simulink model "StSys_StrtCtl"  (R2016b)
settings: configuration reference "CodeGenConfigSet" (kept outside this file)
values from neighbouring files (symbols this model uses):
  Strt_uThresIniMinStrt_C = Calibration.Parameter    [init_StSys_StrtCtl.m]    (also in init_StSys_StrtCtl_SIL.m = Simulink.Parameter)
  StSys_nBlnd_C = Calibration.Parameter    [init_StSys_StrtCtl.m]    (also in init_StSys_StrtCtl_SIL.m = Simulink.Parameter)
  StSys_nThres_C = Calibration.Parameter    [init_StSys_StrtCtl.m]    (also in init_StSys_StrtCtl_SIL.m = Simulink.Parameter)
  StSys_nThresCalc_CUR = Calibration.Parameter    [init_StSys_StrtCtl.m]    (also in init_StSys_StrtCtl_SIL.m = Simulink.Parameter)
  StSys_nThresCalc_CURX = Calibration.Parameter    [init_StSys_StrtCtl.m]    (also in init_StSys_StrtCtl_SIL.m = Simulink.Parameter)
  StSys_stCondActv_C = Calibration.Parameter    [init_StSys_StrtCtl.m]    (also in init_StSys_StrtCtl_SIL.m = Simulink.Parameter)
  StSys_stCondDeactv_C = Calibration.Parameter    [init_StSys_StrtCtl.m]    (also in init_StSys_StrtCtl_SIL.m = Simulink.Parameter)
  StSys_stLogicT50CAN_C = Calibration.Parameter    [init_StSys_StrtCtl.m]    (also in init_StSys_StrtCtl_SIL.m = Simulink.Parameter)
  StSys_stLogicT50EMGCY_C = Calibration.Parameter    [init_StSys_StrtCtl.m]    (also in init_StSys_StrtCtl_SIL.m = Simulink.Parameter)
  StSys_stLogicT50NRM_C = Calibration.Parameter    [init_StSys_StrtCtl.m]    (also in init_StSys_StrtCtl_SIL.m = Simulink.Parameter)
  StSys_stSelectT50CAN_C = Calibration.Parameter    [init_StSys_StrtCtl.m]    (also in init_StSys_StrtCtl_SIL.m = Simulink.Parameter)
  StSys_stSelectT50EMGCY_C = Calibration.Parameter    [init_StSys_StrtCtl.m]    (also in init_StSys_StrtCtl_SIL.m = Simulink.Parameter)
  StSys_stSelectT50NRM_C = Calibration.Parameter    [init_StSys_StrtCtl.m]    (also in init_StSys_StrtCtl_SIL.m = Simulink.Parameter)
  StSys_tiBlnd_C = Calibration.Parameter    [init_StSys_StrtCtl.m]    (also in init_StSys_StrtCtl_SIL.m = Simulink.Parameter)
  StSys_tiStrtON_C = Calibration.Parameter    [init_StSys_StrtCtl.m]    (also in init_StSys_StrtCtl_SIL.m = Simulink.Parameter)
  StSys_vEngCompStrt_C = Calibration.Parameter    [init_StSys_StrtCtl.m]    (also in init_StSys_StrtCtl_SIL.m = Simulink.Parameter)
  StSys_vThresT50CAN_C = Calibration.Parameter    [init_StSys_StrtCtl.m]    (also in init_StSys_StrtCtl_SIL.m = Simulink.Parameter)
  StSys_vThresT50EMGCY_C = Calibration.Parameter    [init_StSys_StrtCtl.m]    (also in init_StSys_StrtCtl_SIL.m = Simulink.Parameter)
  StSys_vThresT50NRM_C = Calibration.Parameter    [init_StSys_StrtCtl.m]    (also in init_StSys_StrtCtl_SIL.m = Simulink.Parameter)
undefined symbols (not defined in the file or in its folder): AirHtState_conv, StSys_StrtCtl_DT, StSys_StrtState_conv
libraries: simulink x201, CXLib x7
(part 1 of 2)
settings Model: Creator=xuxingpei  LastModifiedBy=xuxingpei
settings ConfigSetRef: SourceLocation=Base Workspace

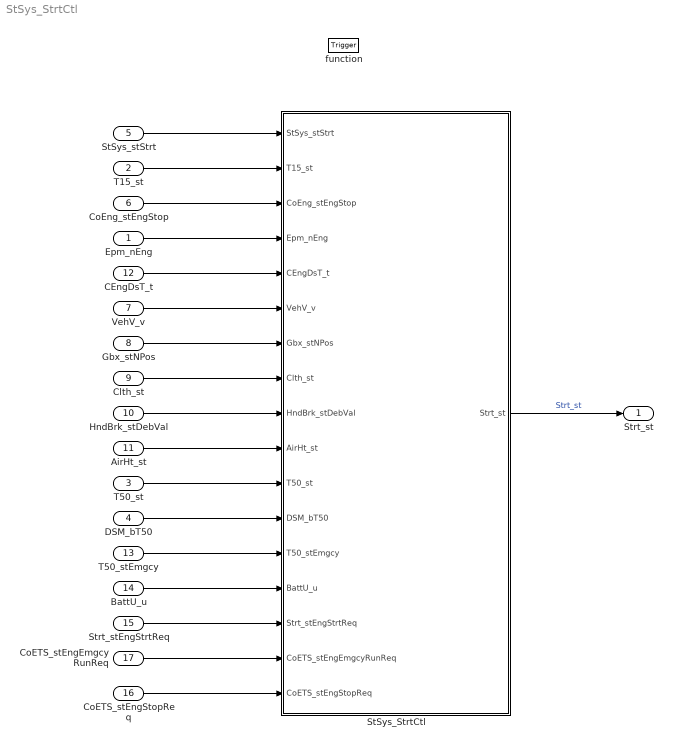
== system StSys_StrtCtl ==
  Epm_nEng : Inport  Tag=rpm  Description=Engine speed  OutMin=0  OutMax=6000  OutDataTypeStr=EngSpeed_rpm
  T15_st : Inport  Description=Terminal 15 status after debouncing  Port=2  OutDataTypeStr=Enum: Switch_conv
  T50_st : Inport  Description=Terminal 50 status after debouncing  Port=3  OutDataTypeStr=Enum: Switch_conv
  DSM_bT50 : Inport  Description=DSM status from T50 switch  Port=4  OutMin=0  OutMax=1  OutDataTypeStr=boolean
  StSys_stStrt : Inport  Description=state of starting system  Port=5  OutDataTypeStr=Enum: StSys_StrtState_conv
  CoEng_stEngStop : Inport  Description=Bit coded output message from engine stop function for low idle, egine shut off and crank control  Port=6  OutMin=0  OutMax=255  OutDataTypeStr=State_uint8
  VehV_v : Inport  Tag=km/h  Description=Vehicle speed  Port=7  OutMin=0  OutMax=250  OutDataTypeStr=VehSpeed_km_h
  Gbx_stNPos : Inport  Description=Gearbox neutral position status signal  Port=8  OutMin=0  OutMax=255  OutDataTypeStr=State_uint8
  Clth_st : Inport  Description=Clutch information  Port=9  OutMin=0  OutMax=255  OutDataTypeStr=State_uint8
  HndBrk_stDebVal : Inport  Description=Debounced value of Hand Brake switch  Port=10  OutMin=0  OutMax=255  OutDataTypeStr=State_uint8
  AirHt_st : Inport  Description=status of AirHeater  Port=11  OutDataTypeStr=Enum: AirHtState_conv
  CEngDsT_t : Inport  Tag=deg  Description=Coolant engine down stream temperature  Port=12  OutMin=-200  OutMax=200  OutDataTypeStr=Temp_deg
  T50_stEmgcy : Inport  Description=Terminal 50 status after debouncing  Port=13  OutMin=0  OutMax=1  OutDataTypeStr=boolean
  BattU_u : Inport  Tag=mv  Description=Battery voltage  Port=14  OutMin=0  OutMax=50000  OutDataTypeStr=Battery_mv
  Strt_stEngStrtReq : Inport  Description=start switch via CAN  Port=15  OutMin=0  OutMax=1  OutDataTypeStr=boolean
  CoETS_stEngStopReq : Inport  Description=Tbox Engine stop request  Port=16  OutMin=0  OutMax=1  OutDataTypeStr=boolean
  CoETS_stEngEmgcyRunReq : Inport  Description=Tbox Engine emergency start request  Port=17  OutMin=0  OutMax=1  OutDataTypeStr=boolean
  function : TriggerPort  TriggerType=function-call  VariantControl=Variant
  StSys_StrtCtl : Subsystem
  Strt_st : Outport  Description=Control signal for the starter relay  OutMin=0  OutMax=1  OutDataTypeStr=boolean
  wires:
  StSys_stStrt/1 -> StSys_StrtCtl/1(StSys_stStrt)
  T15_st/1 -> StSys_StrtCtl/2(T15_st)
  CoEng_stEngStop/1 -> StSys_StrtCtl/3(CoEng_stEngStop)
  Epm_nEng/1 -> StSys_StrtCtl/4(Epm_nEng)
  CEngDsT_t/1 -> StSys_StrtCtl/5(CEngDsT_t)
  VehV_v/1 -> StSys_StrtCtl/6(VehV_v)
  Gbx_stNPos/1 -> StSys_StrtCtl/7(Gbx_stNPos)
  Clth_st/1 -> StSys_StrtCtl/8(Clth_st)
  HndBrk_stDebVal/1 -> StSys_StrtCtl/9(HndBrk_stDebVal)
  AirHt_st/1 -> StSys_StrtCtl/10(AirHt_st)
  T50_st/1 -> StSys_StrtCtl/11(T50_st)
  DSM_bT50/1 -> StSys_StrtCtl/12(DSM_bT50)
  StSys_StrtCtl/1(Strt_st) -> Strt_st/1  "Strt_st"
  T50_stEmgcy/1 -> StSys_StrtCtl/13(T50_stEmgcy)
  BattU_u/1 -> StSys_StrtCtl/14(BattU_u)
  Strt_stEngStrtReq/1 -> StSys_StrtCtl/15(Strt_stEngStrtReq)
  CoETS_stEngStopReq/1 -> StSys_StrtCtl/17(CoETS_stEngStopReq)
  CoETS_stEngEmgcyRunReq/1 -> StSys_StrtCtl/16(CoETS_stEngEmgcyRunReq)

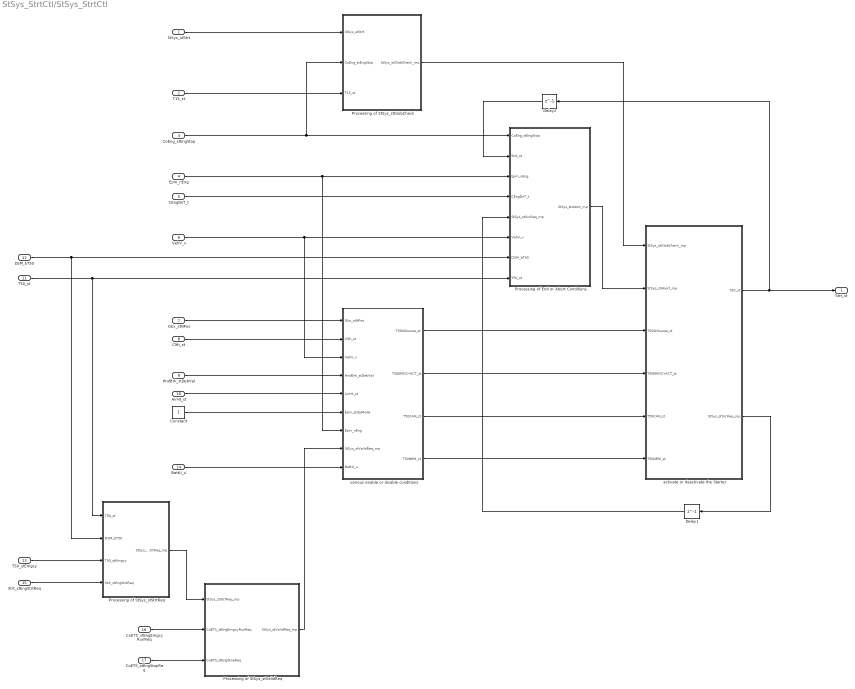
== system StSys_StrtCtl/StSys_StrtCtl ==
  StSys_stStrt : Inport  Description=state of starting system  OutDataTypeStr=Enum: StSys_StrtState_conv
  T15_st : Inport  Description=Terminal 15 status after debouncing  Port=2  OutDataTypeStr=Enum: Switch_conv
  CoEng_stEngStop : Inport  Description=Bit coded output message from engine stop function for low idle, egine shut off and crank control  Port=3  OutMin=0  OutMax=255  OutDataTypeStr=State_uint8
  Epm_nEng : Inport  Tag=rpm  Description=Engine speed  Port=4  OutMin=0  OutMax=6000  OutDataTypeStr=EngSpeed_rpm
  CEngDsT_t : Inport  Tag=deg  Description=Coolant engine down stream temperature  Port=5  OutMin=-200  OutMax=200  OutDataTypeStr=Temp_deg
  VehV_v : Inport  Tag=km/h  Description=Vehicle speed  Port=6  OutMin=0  OutMax=250  OutDataTypeStr=VehSpeed_km_h
  Gbx_stNPos : Inport  Description=Gearbox neutral position status signal  Port=7  OutMin=0  OutMax=255  OutDataTypeStr=State_uint8
  Clth_st : Inport  Description=Clutch information  Port=8  OutMin=0  OutMax=255  OutDataTypeStr=State_uint8
  HndBrk_stDebVal : Inport  Description=Debounced value of Hand Brake switch  Port=9  OutMin=0  OutMax=255  OutDataTypeStr=State_uint8
  AirHt_st : Inport  Description=status of AirHeater  Port=10  OutDataTypeStr=Enum: AirHtState_conv
  T50_st : Inport  Description=Terminal 15 status after debouncing  Port=11  OutDataTypeStr=Enum: Switch_conv
  DSM_bT50 : Inport  Description=DSM status from T50 switch  Port=12  OutMin=0  OutMax=1  OutDataTypeStr=boolean
  T50_stEmgcy : Inport  Port=13
  BattU_u : Inport  Port=14
  Strt_stEngStrtReq : Inport  Description=start switch via CAN  Port=15  OutMin=0  OutMax=1  OutDataTypeStr=boolean
  CoETS_stEngEmgcyRunReq : Inport  Port=16
  CoETS_stEngStopReq : Inport  Port=17
  Constant : Constant  OutDataTypeStr=boolean
  Delay1 : Delay  DelayLength=1  InitialCondition=0
  Delay2 : Delay  DelayLength=1  InitialCondition=0
  Processing of End or Abort Conditions : Subsystem
  Processing of StSys_stGlobCheck : Subsystem
  Processing of StSys_stStrtReq : Subsystem
  Processing of StSys_stValidReq : Subsystem
  activate or deactivate the Starter : Subsystem
  various enable or disable conditions : Subsystem
  Strt_st : Outport  Description=Control signal for the starter relay  OutMin=0  OutMax=1  OutDataTypeStr=boolean
  wires:
  activate or deactivate the Starter/1(Strt_st) -> Delay2/1, Strt_st/1
  CoEng_stEngStop/1 -> Processing of StSys_stGlobCheck/2(CoEng_stEngStop), Processing of End or Abort Conditions/1(CoEng_stEngStop)
  Constant/1 -> various enable or disable conditions/6(Epm_stOpMode)
  DSM_bT50/1 -> Processing of StSys_stStrtReq/2(DSM_bT50), Processing of End or Abort Conditions/7(DSM_bT50)
  Processing of StSys_stStrtReq/1(StSys_stStrtReq_mp) -> Processing of StSys_stValidReq/1(StSys_stStrtReq_mp)
  Epm_nEng/1 -> various enable or disable conditions/7(Epm_nEng), Processing of End or Abort Conditions/3(Epm_nEng)
  T50_stEmgcy/1 -> Processing of StSys_stStrtReq/3(T50_stEmgcy)
  HndBrk_stDebVal/1 -> various enable or disable conditions/4(HndBrk_stDebVal)
  StSys_stStrt/1 -> Processing of StSys_stGlobCheck/1(StSys_stStrt)
  Gbx_stNPos/1 -> various enable or disable conditions/1(Gbx_stNPos)
  T50_st/1 -> Processing of StSys_stStrtReq/1(T50_st), Processing of End or Abort Conditions/8(T50_st)
  AirHt_st/1 -> various enable or disable conditions/5(AirHt_st)
  Clth_st/1 -> various enable or disable conditions/2(Clth_st)
  Processing of StSys_stValidReq/1(StSys_stValidReq_mp) -> various enable or disable conditions/8(StSys_stValidReq_mp)
  various enable or disable conditions/1(T50StSourse_st) -> activate or deactivate the Starter/3(T50StSourse_st)
  T15_st/1 -> Processing of StSys_stGlobCheck/3(T15_st)
  VehV_v/1 -> various enable or disable conditions/3(VehV_v), Processing of End or Abort Conditions/6(VehV_v)
  CEngDsT_t/1 -> Processing of End or Abort Conditions/4(CEngDsT_t)
  BattU_u/1 -> various enable or disable conditions/9(BattU_u)
  various enable or disable conditions/2(T50EMGCYACT_st) -> activate or deactivate the Starter/4(T50EMGCYACT_st)
  Processing of StSys_stGlobCheck/1(StSys_stGlobCheck_mp) -> activate or deactivate the Starter/1(StSys_stGlobCheck_mp)
  Processing of End or Abort Conditions/1(StSys_stAbort_mp) -> activate or deactivate the Starter/2(StSys_stAbort_mp)
  activate or deactivate the Starter/2(StSys_stSrcReq_mp) -> Delay1/1
  Delay1/1 -> Processing of End or Abort Conditions/5(StSys_stSrcReq_mp)
  Delay2/1 -> Processing of End or Abort Conditions/2(Strt_st)
  various enable or disable conditions/3(T50CAN_st) -> activate or deactivate the Starter/5(T50CAN_st)
  Strt_stEngStrtReq/1 -> Processing of StSys_stStrtReq/4(Strt_stEngStrtReq)
  various enable or disable conditions/4(T50NRM_st) -> activate or deactivate the Starter/6(T50NRM_st)
  CoETS_stEngEmgcyRunReq/1 -> Processing of StSys_stValidReq/2(CoETS_stEngEmgcyRunReq)
  CoETS_stEngStopReq/1 -> Processing of StSys_stValidReq/3(CoETS_stEngStopReq)

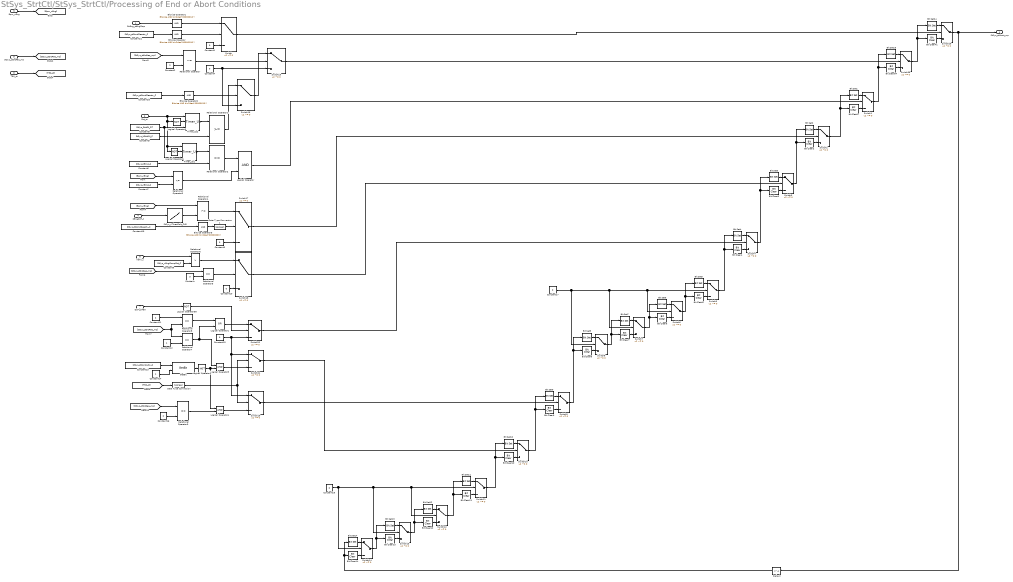
== system StSys_StrtCtl/StSys_StrtCtl/Processing of End or Abort Conditions ==
  CoEng_stEngStop : Inport
  Strt_st : Inport  Port=2
  Epm_nEng : Inport  Port=3
  CEngDsT_t : Inport  Port=4
  StSys_stSrcReq_mp : Inport  Port=5
  VehV_v : Inport  Port=6
  DSM_bT50 : Inport  Port=7
  T50_st : Inport  Port=8
  Bit Clear1 : simulink/Logic and Bit Operations/Bit Clear  iBit=2
  Bit Clear10 : simulink/Logic and Bit Operations/Bit Clear  iBit=11
  Bit Clear11 : simulink/Logic and Bit Operations/Bit Clear  iBit=12
  Bit Clear12 : simulink/Logic and Bit Operations/Bit Clear  iBit=13
  Bit Clear13 : simulink/Logic and Bit Operations/Bit Clear  iBit=14
  Bit Clear14 : simulink/Logic and Bit Operations/Bit Clear  iBit=15
  Bit Clear2 : simulink/Logic and Bit Operations/Bit Clear  iBit=3
  Bit Clear3 : simulink/Logic and Bit Operations/Bit Clear  iBit=4
  Bit Clear4 : simulink/Logic and Bit Operations/Bit Clear  iBit=5
  Bit Clear41 : simulink/Logic and Bit Operations/Bit Clear  iBit=0
  Bit Clear5 : simulink/Logic and Bit Operations/Bit Clear  iBit=6
  Bit Clear54 : simulink/Logic and Bit Operations/Bit Clear  iBit=1
  Bit Clear6 : simulink/Logic and Bit Operations/Bit Clear  iBit=7
  Bit Clear7 : simulink/Logic and Bit Operations/Bit Clear  iBit=8
  Bit Clear8 : simulink/Logic and Bit Operations/Bit Clear  iBit=9
  Bit Clear9 : simulink/Logic and Bit Operations/Bit Clear  iBit=10
  Bit Set1 : simulink/Logic and Bit Operations/Bit Set  iBit=2
  Bit Set10 : simulink/Logic and Bit Operations/Bit Set  iBit=11
  Bit Set11 : simulink/Logic and Bit Operations/Bit Set  iBit=12
  Bit Set12 : simulink/Logic and Bit Operations/Bit Set  iBit=13
  Bit Set13 : simulink/Logic and Bit Operations/Bit Set  iBit=14
  Bit Set14 : simulink/Logic and Bit Operations/Bit Set  iBit=15
  Bit Set18 : simulink/Logic and Bit Operations/Bit Set  iBit=1
  Bit Set2 : simulink/Logic and Bit Operations/Bit Set  iBit=3
  Bit Set24 : simulink/Logic and Bit Operations/Bit Set  iBit=0
  Bit Set3 : simulink/Logic and Bit Operations/Bit Set  iBit=4
  Bit Set4 : simulink/Logic and Bit Operations/Bit Set  iBit=5
  Bit Set5 : simulink/Logic and Bit Operations/Bit Set  iBit=6
  Bit Set6 : simulink/Logic and Bit Operations/Bit Set  iBit=7
  Bit Set7 : simulink/Logic and Bit Operations/Bit Set  iBit=8
  Bit Set8 : simulink/Logic and Bit Operations/Bit Set  iBit=9
  Bit Set9 : simulink/Logic and Bit Operations/Bit Set  iBit=10
  Bitwise Operator : simulink/Logic and Bit Operations/Bitwise Operator  logicop=AND  UseBitMask=on  BitMask=bin2dec('00000100')  BitMaskRealWorld=Stored Integer
  Bitwise Operator1 : simulink/Logic and Bit Operations/Bitwise Operator  logicop=AND  UseBitMask=on  BitMask=bin2dec('00000010')  BitMaskRealWorld=Stored Integer
  Bitwise Operator2 : simulink/Logic and Bit Operations/Bitwise Operator  logicop=AND  UseBitMask=on  BitMask=bin2dec('00000010')  BitMaskRealWorld=Stored Integer
  Bitwise Operator3 : simulink/Logic and Bit Operations/Bitwise Operator  logicop=AND  UseBitMask=on  BitMask=bin2dec('00000001')  BitMaskRealWorld=Stored Integer
  Constant : Constant  Value=3  OutDataTypeStr=Inherit: Inherit via back propagation
  Constant{1,3..4,10,15} (5 alike) : Constant  Value=0  OutDataTypeStr=Inherit: Inherit via back propagation
  Constant11 : Constant  Value=2  OutDataTypeStr=Inherit: Inherit via back propagation
  Constant12 : Constant  OutDataTypeStr=Inherit: Inherit via back propagation
  Constant13 : Constant  Value=StSys_stCondActv_C
  Constant14 : Constant  OutDataTypeStr=Inherit: Inherit via back propagation
  Constant16 : Constant  Value=2  OutDataTypeStr=Inherit: Inherit via back propagation
  Constant17 : Constant  Value=0  OutDataTypeStr=boolean
  Constant18 : Constant  Value=0  OutDataTypeStr=boolean
  Constant19 : Constant  Value=StSys_stCondDeactv_C
  Constant2 : Constant  Value=2  OutDataTypeStr=Inherit: Inherit via back propagation
  Constant20 : Constant  Value=StSys_stCondDeactv_C
  Constant21 : Constant  Value=StSys_stCondDeactv_C
  Constant5 : Constant  Value=StSys_tiStrtON_C
  Constant6 : Constant  Value=StSys_tiBlnd_C
  Constant7 : Constant  Value=StSys_nBlnd_C
  Constant8 : Constant  Value=StSys_StrtCtl_DT
  Constant9 : Constant  Value=StSys_vEngCompStrt_C
  Data Type Conversion : DataTypeConversion  OutDataTypeStr=boolean
  Data Type Conversion1 : DataTypeConversion  OutDataTypeStr=boolean
  Delay2 : Delay  DelayLength=1  InitialCondition=0
  GetBit : CXLib/GetBit  dataTypeString=uint16  dataLength=0
      settings: AttributesFormatString=Get bit from %<dataTypeString>
  Logical Operator : Logic  OutDataTypeStr=boolean
  Logical Operator1 : Logic  Operator=OR  AllPortsSameDT=off  OutDataTypeStr=boolean
  Logical Operator{2,5..6,38} (4 alike) : Logic  Operator=NOT  AllPortsSameDT=off  OutDataTypeStr=boolean
  Logical Operator3 : Logic  AllPortsSameDT=off  OutDataTypeStr=boolean
  Logical Operator4 : Logic  AllPortsSameDT=off  OutDataTypeStr=boolean
  Relational Operator : RelationalOperator  Operator=~=  OutDataTypeStr=boolean  RndMeth=Simplest  InputSameDT=on
  Relational Operator1 : RelationalOperator  OutDataTypeStr=boolean  RndMeth=Simplest
  Relational Operator2 : RelationalOperator  OutDataTypeStr=boolean  RndMeth=Simplest
  Relational Operator3 : RelationalOperator  Operator=<=  OutDataTypeStr=boolean  RndMeth=Simplest
  Relational Operator4 : RelationalOperator  OutDataTypeStr=boolean  RndMeth=Simplest
  Relational Operator{5,7..9} (4 alike) : RelationalOperator  Operator===  OutDataTypeStr=boolean  RndMeth=Simplest  InputSameDT=on
  Relational Operator6 : RelationalOperator  Operator=>  OutDataTypeStr=boolean  RndMeth=Simplest
  StSys_nThresCalc_CUR : Lookup_n-D  NumberOfTableDimensions=1  BreakpointsForDimension1=StSys_nThresCalc_CURX  BreakpointsForDimension1DataTypeStr=Temp_deg  IndexSearchMethod=Linear search  Table=StSys_nThresCalc_CUR  TableDataTypeStr=EngSpeed_rpm  ExtrapMethod=Clip  InternalRulePriority=Speed  OutDataTypeStr=EngSpeed_rpm  RndMeth=Simplest  InputSameDT=on
  Switch{,1..14,16..18,20,29,36} (21 alike) : Switch  Criteria=u2 ~= 0  InputSameDT=on
  Switch15 : Switch  Criteria=u2 ~= 0
  Switch19 : Switch  Criteria=u2 ~= 0
  Switch21 : Switch  Criteria=u2 ~= 0
  Timer_Up1 : CXLib/Timer_Up
  Timer_Up2 : CXLib/Timer_Up
  StSys_stAbort_mp : Outport
  wires:
  Switch29/1 -> Delay2/1, StSys_stAbort_mp/1  "StSys_stAbort_mp"
  Bit Set24/1 -> Switch29/1
  Bit Clear41/1 -> Switch29/3
  Delay2/1 -> Bit Clear14/1, Bit Set14/1
  Switch36/1 -> Bit Clear41/1, Bit Set24/1
  Bit Set18/1 -> Switch36/1
  Bit Clear54/1 -> Switch36/3
  Switch1/1 -> Bit Set18/1, Bit Clear54/1
  Bit Set1/1 -> Switch1/1
  Bit Clear1/1 -> Switch1/3
  Switch2/1 -> Bit Set1/1, Bit Clear1/1
  Bit Set2/1 -> Switch2/1
  Bit Clear2/1 -> Switch2/3
  Switch3/1 -> Bit Clear2/1, Bit Set2/1
  Bit Set3/1 -> Switch3/1
  Bit Clear3/1 -> Switch3/3
  Switch4/1 -> Bit Set3/1, Bit Clear3/1
  Bit Set4/1 -> Switch4/1
  Bit Clear4/1 -> Switch4/3
  Switch5/1 -> Bit Set4/1, Bit Clear4/1
  Bit Set5/1 -> Switch5/1
  Bit Clear5/1 -> Switch5/3
  Switch6/1 -> Bit Set5/1, Bit Clear5/1
  Bit Set6/1 -> Switch6/1
  Bit Clear6/1 -> Switch6/3
  Switch7/1 -> Bit Set6/1, Bit Clear6/1
  Bit Set7/1 -> Switch7/1
  Bit Clear7/1 -> Switch7/3
  Switch8/1 -> Bit Set7/1, Bit Clear7/1
  Bit Set8/1 -> Switch8/1
  Bit Clear8/1 -> Switch8/3
  Switch9/1 -> Bit Set8/1, Bit Clear8/1
  Bit Set9/1 -> Switch9/1
  Bit Clear9/1 -> Switch9/3
  Switch10/1 -> Bit Set9/1, Bit Clear9/1
  Bit Set10/1 -> Switch10/1
  Bit Clear10/1 -> Switch10/3
  Switch11/1 -> Bit Clear10/1, Bit Set10/1
  Bit Set11/1 -> Switch11/1
  Bit Clear11/1 -> Switch11/3
  Switch12/1 -> Bit Set11/1, Bit Clear11/1
  Bit Set12/1 -> Switch12/1
  Bit Clear12/1 -> Switch12/3
  Switch13/1 -> Bit Set12/1, Bit Clear12/1
  Bit Set13/1 -> Switch13/1
  Bit Clear13/1 -> Switch13/3
  Switch14/1 -> Bit Set13/1, Bit Clear13/1
  Bit Set14/1 -> Switch14/1
  Bit Clear14/1 -> Switch14/3
  Bitwise Operator/1 -> Switch/2
  CoEng_stEngStop/1 -> Bitwise Operator1/1
  Constant21/1 -> Bitwise Operator/1
  [StSys_stSrcReq_mp] -> Relational Operator/1
  Constant2/1 -> Relational Operator/2
  Relational Operator/1 -> Switch15/2
  Constant20/1 -> Bitwise Operator2/1
  Bitwise Operator2/1 -> Switch16/2
  Constant4/1 -> Switch16/3, Switch15/3
  Timer_Up1/1 -> Relational Operator2/1
  Constant6/1 -> Relational Operator2/2
  Timer_Up2/1 -> Relational Operator1/1
  Constant5/1 -> Relational Operator1/2
  [Epm_nEng] -> Relational Operator3/1
  Constant7/1 -> Relational Operator3/2
  Relational Operator2/1 -> Logical Operator/1
  Relational Operator3/1 -> Logical Operator/2
  Epm_nEng/1 -> [Epm_nEng]
  Constant19/1 -> Bitwise Operator3/1
  CEngDsT_t/1 -> StSys_nThresCalc_CUR/1
  StSys_nThresCalc_CUR/1 -> Relational Operator4/2
  [Epm_nEng] -> Relational Operator4/1
  Bitwise Operator3/1 -> Data Type Conversion1/1
  StSys_stSrcReq_mp/1 -> [StSys_stSrcReq_mp]
  [StSys_stSrcReq_mp] -> Relational Operator5/1
  Constant/1 -> Relational Operator5/2
  VehV_v/1 -> Relational Operator6/1
  Constant9/1 -> Relational Operator6/2
  Relational Operator5/1 -> Switch18/2
  DSM_bT50/1 -> Logical Operator38/1
  Logical Operator38/1 -> Switch20/2
  Relational Operator8/1 -> Logical Operator1/1
  Relational Operator7/1 -> Logical Operator1/2, Logical Operator3/1
  [StSys_stSrcReq_mp] -> Relational Operator8/2, Relational Operator7/1
  Constant11/1 -> Relational Operator8/1
  Constant12/1 -> Relational Operator7/2
  Constant13/1 -> GetBit/1
  Constant14/1 -> GetBit/2
  GetBit/1 -> Logical Operator2/1
  Logical Operator2/1 -> Logical Operator4/1, Logical Operator3/2
  T50_st/1 -> [T50_st]
  [T50_st] -> Data Type Conversion/1
  Constant15/1 -> Switch19/1, Switch21/1, Switch20/3
  [StSys_stSrcReq_mp] -> Relational Operator9/1
  Constant16/1 -> Relational Operator9/2
  Relational Operator9/1 -> Logical Operator4/2
  Switch/1 -> Switch29/2
  Switch15/1 -> Switch36/2
  Logical Operator/1 -> Switch1/2
  Constant17/1 -> Switch8/2, Switch7/2, Switch6/2, Switch5/2
  Constant18/1 -> Switch14/2, Switch13/2, Switch12/2, Switch11/2
  Switch21/1 -> Switch10/2
  Switch19/1 -> Switch9/2
  Constant8/1 -> Timer_Up2/3, Timer_Up1/3
  Switch17/1 -> Switch2/2
  Switch18/1 -> Switch3/2
  Switch20/1 -> Switch4/2
  Logical Operator4/1 -> Switch19/3
  Logical Operator3/1 -> Switch21/3
  Logical Operator1/1 -> Switch20/1
  Relational Operator6/1 -> Switch18/1
  Constant10/1 -> Switch18/3
  Relational Operator4/1 -> Switch17/1
  Constant3/1 -> Switch17/3
  Relational Operator1/1 -> Switch16/1
  Switch16/1 -> Switch15/1
  Bitwise Operator1/1 -> Switch/1
  Constant1/1 -> Switch/3
  Data Type Conversion/1 -> Switch19/2, Switch21/2
  Data Type Conversion1/1 -> Switch17/2
  Logical Operator5/1 -> Timer_Up2/2
  Logical Operator6/1 -> Timer_Up1/2
  Strt_st/1 -> Timer_Up2/1, Logical Operator5/1, Logical Operator6/1, Timer_Up1/1

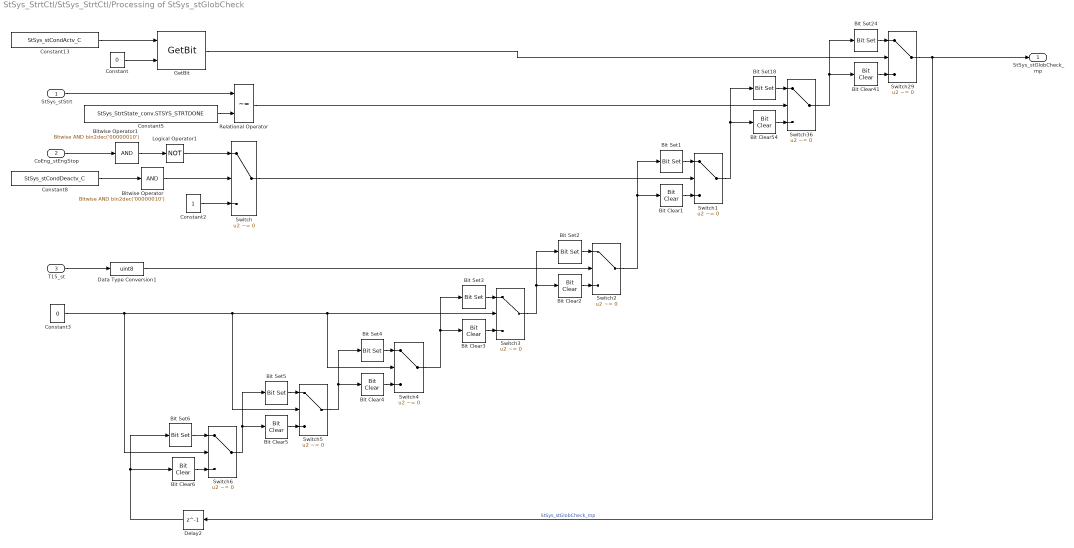
== system StSys_StrtCtl/StSys_StrtCtl/Processing of StSys_stGlobCheck ==
  StSys_stStrt : Inport
  CoEng_stEngStop : Inport  Port=2
  T15_st : Inport  Port=3
  Bit Clear1 : simulink/Logic and Bit Operations/Bit Clear  iBit=2
  Bit Clear2 : simulink/Logic and Bit Operations/Bit Clear  iBit=3
  Bit Clear3 : simulink/Logic and Bit Operations/Bit Clear  iBit=4
  Bit Clear4 : simulink/Logic and Bit Operations/Bit Clear  iBit=5
  Bit Clear41 : simulink/Logic and Bit Operations/Bit Clear  iBit=0
  Bit Clear5 : simulink/Logic and Bit Operations/Bit Clear  iBit=6
  Bit Clear54 : simulink/Logic and Bit Operations/Bit Clear  iBit=1
  Bit Clear6 : simulink/Logic and Bit Operations/Bit Clear  iBit=7
  Bit Set1 : simulink/Logic and Bit Operations/Bit Set  iBit=2
  Bit Set18 : simulink/Logic and Bit Operations/Bit Set  iBit=1
  Bit Set2 : simulink/Logic and Bit Operations/Bit Set  iBit=3
  Bit Set24 : simulink/Logic and Bit Operations/Bit Set  iBit=0
  Bit Set3 : simulink/Logic and Bit Operations/Bit Set  iBit=4
  Bit Set4 : simulink/Logic and Bit Operations/Bit Set  iBit=5
  Bit Set5 : simulink/Logic and Bit Operations/Bit Set  iBit=6
  Bit Set6 : simulink/Logic and Bit Operations/Bit Set  iBit=7
  Bitwise Operator : simulink/Logic and Bit Operations/Bitwise Operator  logicop=AND  UseBitMask=on  BitMask=bin2dec('00000010')  BitMaskRealWorld=Stored Integer
  Bitwise Operator1 : simulink/Logic and Bit Operations/Bitwise Operator  logicop=AND  UseBitMask=on  BitMask=bin2dec('00000010')  BitMaskRealWorld=Stored Integer
  Constant : Constant  Value=0  OutDataTypeStr=uint8
  Constant13 : Constant  Value=StSys_stCondActv_C
  Constant2 : Constant  OutDataTypeStr=Inherit: Inherit via back propagation
  Constant3 : Constant  Value=0  OutDataTypeStr=boolean
  Constant5 : Constant  Value=StSys_StrtState_conv.STSYS_STRTDONE
  Constant8 : Constant  Value=StSys_stCondDeactv_C
  Data Type Conversion1 : DataTypeConversion  OutDataTypeStr=uint8
  Delay2 : Delay  DelayLength=1  InitialCondition=0
  GetBit : CXLib/GetBit  dataTypeString=uint16  dataLength=0
      settings: AttributesFormatString=Get bit from %<dataTypeString>
  Logical Operator1 : Logic  Operator=NOT  AllPortsSameDT=off  OutDataTypeStr=boolean
  Relational Operator : RelationalOperator  Operator=~=  OutDataTypeStr=boolean  RndMeth=Simplest
  Switch{,1..6,29,36} (9 alike) : Switch  Criteria=u2 ~= 0  InputSameDT=on
  StSys_stGlobCheck_mp : Outport
  wires:
  Switch29/1 -> StSys_stGlobCheck_mp/1, Delay2/1  "StSys_stGlobCheck_mp"
  Bit Set24/1 -> Switch29/1
  Bit Clear41/1 -> Switch29/3
  Switch36/1 -> Bit Clear41/1, Bit Set24/1
  Bit Set18/1 -> Switch36/1
  Bit Clear54/1 -> Switch36/3
  Switch1/1 -> Bit Set18/1, Bit Clear54/1
  Bit Set1/1 -> Switch1/1
  Bit Clear1/1 -> Switch1/3
  Switch2/1 -> Bit Set1/1, Bit Clear1/1
  Bit Set2/1 -> Switch2/1
  Bit Clear2/1 -> Switch2/3
  Switch3/1 -> Bit Clear2/1, Bit Set2/1
  Bit Set3/1 -> Switch3/1
  Bit Clear3/1 -> Switch3/3
  Switch4/1 -> Bit Set3/1, Bit Clear3/1
  Bit Set4/1 -> Switch4/1
  Bit Clear4/1 -> Switch4/3
  Switch5/1 -> Bit Set4/1, Bit Clear4/1
  Bit Set5/1 -> Switch5/1
  Bit Clear5/1 -> Switch5/3
  Switch6/1 -> Bit Set5/1, Bit Clear5/1
  Bit Set6/1 -> Switch6/1
  Bit Clear6/1 -> Switch6/3
  Delay2/1 -> Bit Clear6/1, Bit Set6/1
  Constant8/1 -> Bitwise Operator/1
  Constant13/1 -> GetBit/1
  Constant/1 -> GetBit/2
  GetBit/1 -> Switch29/2
  Constant5/1 -> Relational Operator/2
  Bitwise Operator/1 -> Switch/2
  CoEng_stEngStop/1 -> Bitwise Operator1/1
  Bitwise Operator1/1 -> Logical Operator1/1
  Relational Operator/1 -> Switch36/2
  Switch/1 -> Switch1/2
  T15_st/1 -> Data Type Conversion1/1
  Constant3/1 -> Switch6/2, Switch5/2, Switch4/2, Switch3/2
  Logical Operator1/1 -> Switch/1
  Constant2/1 -> Switch/3
  StSys_stStrt/1 -> Relational Operator/1
  Data Type Conversion1/1 -> Switch2/2

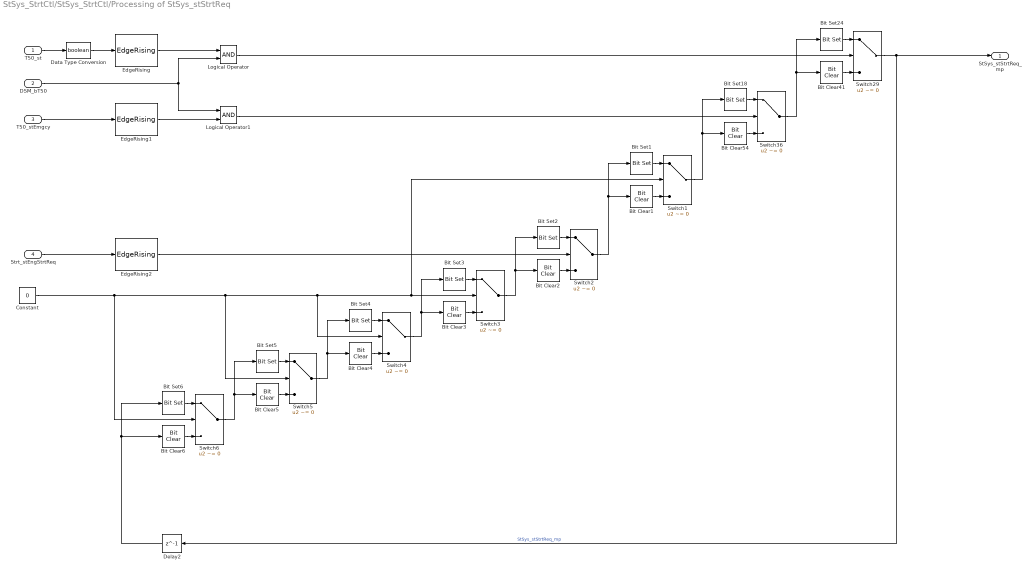
== system StSys_StrtCtl/StSys_StrtCtl/Processing of StSys_stStrtReq ==
  T50_st : Inport
  DSM_bT50 : Inport  Port=2
  T50_stEmgcy : Inport  Port=3
  Strt_stEngStrtReq : Inport  Port=4
  Bit Clear1 : simulink/Logic and Bit Operations/Bit Clear  iBit=2
  Bit Clear2 : simulink/Logic and Bit Operations/Bit Clear  iBit=3
  Bit Clear3 : simulink/Logic and Bit Operations/Bit Clear  iBit=4
  Bit Clear4 : simulink/Logic and Bit Operations/Bit Clear  iBit=5
  Bit Clear41 : simulink/Logic and Bit Operations/Bit Clear  iBit=0
  Bit Clear5 : simulink/Logic and Bit Operations/Bit Clear  iBit=6
  Bit Clear54 : simulink/Logic and Bit Operations/Bit Clear  iBit=1
  Bit Clear6 : simulink/Logic and Bit Operations/Bit Clear  iBit=7
  Bit Set1 : simulink/Logic and Bit Operations/Bit Set  iBit=2
  Bit Set18 : simulink/Logic and Bit Operations/Bit Set  iBit=1
  Bit Set2 : simulink/Logic and Bit Operations/Bit Set  iBit=3
  Bit Set24 : simulink/Logic and Bit Operations/Bit Set  iBit=0
  Bit Set3 : simulink/Logic and Bit Operations/Bit Set  iBit=4
  Bit Set4 : simulink/Logic and Bit Operations/Bit Set  iBit=5
  Bit Set5 : simulink/Logic and Bit Operations/Bit Set  iBit=6
  Bit Set6 : simulink/Logic and Bit Operations/Bit Set  iBit=7
  Constant : Constant  Value=0  OutDataTypeStr=boolean
  Data Type Conversion : DataTypeConversion  OutDataTypeStr=boolean
  Delay2 : Delay  DelayLength=1  InitialCondition=0
  EdgeRising : CXLib/EdgeRising
  EdgeRising1 : CXLib/EdgeRising
  EdgeRising2 : CXLib/EdgeRising
  Logical Operator : Logic  AllPortsSameDT=off  OutDataTypeStr=boolean
  Logical Operator1 : Logic  AllPortsSameDT=off  OutDataTypeStr=boolean
  Switch{1..6,29,36} (8 alike) : Switch  Criteria=u2 ~= 0  InputSameDT=on
  StSys_stStrtReq_mp : Outport
  wires:
  Switch29/1 -> StSys_stStrtReq_mp/1, Delay2/1  "StSys_stStrtReq_mp"
  Bit Set24/1 -> Switch29/1
  Bit Clear41/1 -> Switch29/3
  Switch36/1 -> Bit Clear41/1, Bit Set24/1
  Bit Set18/1 -> Switch36/1
  Bit Clear54/1 -> Switch36/3
  Switch1/1 -> Bit Set18/1, Bit Clear54/1
  Bit Set1/1 -> Switch1/1
  Bit Clear1/1 -> Switch1/3
  Switch2/1 -> Bit Set1/1, Bit Clear1/1
  Bit Set2/1 -> Switch2/1
  Bit Clear2/1 -> Switch2/3
  Switch3/1 -> Bit Clear2/1, Bit Set2/1
  Bit Set3/1 -> Switch3/1
  Bit Clear3/1 -> Switch3/3
  Switch4/1 -> Bit Set3/1, Bit Clear3/1
  Bit Set4/1 -> Switch4/1
  Bit Clear4/1 -> Switch4/3
  Switch5/1 -> Bit Set4/1, Bit Clear4/1
  Bit Set5/1 -> Switch5/1
  Bit Clear5/1 -> Switch5/3
  Switch6/1 -> Bit Set5/1, Bit Clear5/1
  Bit Set6/1 -> Switch6/1
  Bit Clear6/1 -> Switch6/3
  Delay2/1 -> Bit Clear6/1, Bit Set6/1
  T50_st/1 -> Data Type Conversion/1
  EdgeRising/1 -> Logical Operator/1
  DSM_bT50/1 -> Logical Operator1/1, Logical Operator/2
  EdgeRising1/1 -> Logical Operator1/2
  Constant/1 -> Switch1/2, Switch3/2, Switch4/2, Switch5/2, Switch6/2
  Logical Operator1/1 -> Switch36/2
  Logical Operator/1 -> Switch29/2
  Data Type Conversion/1 -> EdgeRising/1
  T50_stEmgcy/1 -> EdgeRising1/1
  Strt_stEngStrtReq/1 -> EdgeRising2/1
  EdgeRising2/1 -> Switch2/2

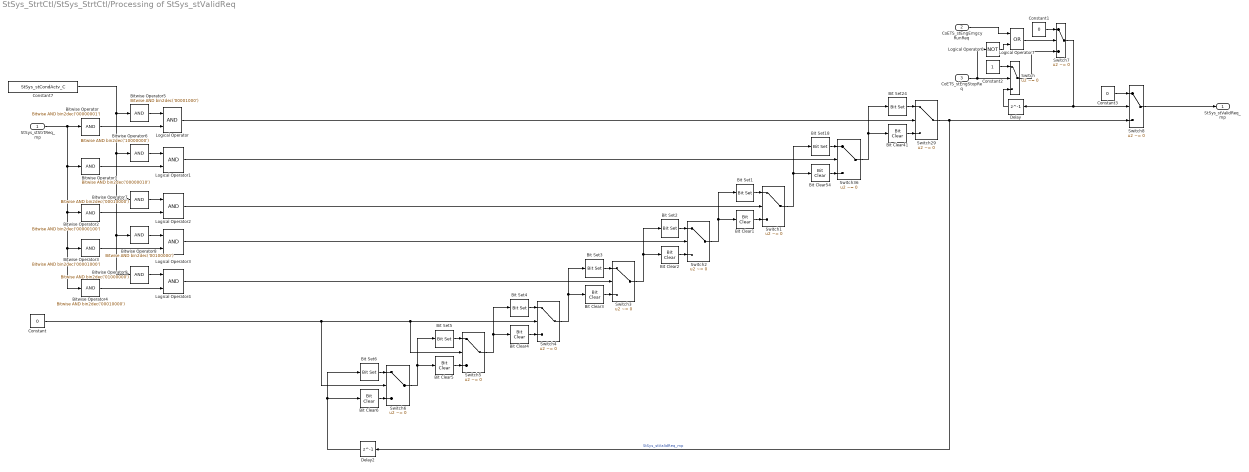
== system StSys_StrtCtl/StSys_StrtCtl/Processing of StSys_stValidReq ==
  StSys_stStrtReq_mp : Inport
  CoETS_stEngEmgcyRunReq : Inport  Port=2
  CoETS_stEngStopReq : Inport  Port=3
  Bit Clear1 : simulink/Logic and Bit Operations/Bit Clear  iBit=2
  Bit Clear2 : simulink/Logic and Bit Operations/Bit Clear  iBit=3
  Bit Clear3 : simulink/Logic and Bit Operations/Bit Clear  iBit=4
  Bit Clear4 : simulink/Logic and Bit Operations/Bit Clear  iBit=5
  Bit Clear41 : simulink/Logic and Bit Operations/Bit Clear  iBit=0
  Bit Clear5 : simulink/Logic and Bit Operations/Bit Clear  iBit=6
  Bit Clear54 : simulink/Logic and Bit Operations/Bit Clear  iBit=1
  Bit Clear6 : simulink/Logic and Bit Operations/Bit Clear  iBit=7
  Bit Set1 : simulink/Logic and Bit Operations/Bit Set  iBit=2
  Bit Set18 : simulink/Logic and Bit Operations/Bit Set  iBit=1
  Bit Set2 : simulink/Logic and Bit Operations/Bit Set  iBit=3
  Bit Set24 : simulink/Logic and Bit Operations/Bit Set  iBit=0
  Bit Set3 : simulink/Logic and Bit Operations/Bit Set  iBit=4
  Bit Set4 : simulink/Logic and Bit Operations/Bit Set  iBit=5
  Bit Set5 : simulink/Logic and Bit Operations/Bit Set  iBit=6
  Bit Set6 : simulink/Logic and Bit Operations/Bit Set  iBit=7
  Bitwise Operator : simulink/Logic and Bit Operations/Bitwise Operator  logicop=AND  UseBitMask=on  BitMask=bin2dec('00000001')  BitMaskRealWorld=Stored Integer
  Bitwise Operator1 : simulink/Logic and Bit Operations/Bitwise Operator  logicop=AND  UseBitMask=on  BitMask=bin2dec('00000010')  BitMaskRealWorld=Stored Integer
  Bitwise Operator2 : simulink/Logic and Bit Operations/Bitwise Operator  logicop=AND  UseBitMask=on  BitMask=bin2dec('00000100')  BitMaskRealWorld=Stored Integer
  Bitwise Operator3 : simulink/Logic and Bit Operations/Bitwise Operator  logicop=AND  UseBitMask=on  BitMask=bin2dec('00001000')  BitMaskRealWorld=Stored Integer
  Bitwise Operator4 : simulink/Logic and Bit Operations/Bitwise Operator  logicop=AND  UseBitMask=on  BitMask=bin2dec('00010000')  BitMaskRealWorld=Stored Integer
  Bitwise Operator5 : simulink/Logic and Bit Operations/Bitwise Operator  logicop=AND  UseBitMask=on  BitMask=bin2dec('00001000')  BitMaskRealWorld=Stored Integer
  Bitwise Operator6 : simulink/Logic and Bit Operations/Bitwise Operator  logicop=AND  UseBitMask=on  BitMask=bin2dec('10000000')  BitMaskRealWorld=Stored Integer
  Bitwise Operator7 : simulink/Logic and Bit Operations/Bitwise Operator  logicop=AND  UseBitMask=on  BitMask=bin2dec('00010000')  BitMaskRealWorld=Stored Integer
  Bitwise Operator8 : simulink/Logic and Bit Operations/Bitwise Operator  logicop=AND  UseBitMask=on  BitMask=bin2dec('00100000')  BitMaskRealWorld=Stored Integer
  Bitwise Operator9 : simulink/Logic and Bit Operations/Bitwise Operator  logicop=AND  UseBitMask=on  BitMask=bin2dec('01000000')  BitMaskRealWorld=Stored Integer
  Constant : Constant  Value=0  OutDataTypeStr=boolean
  Constant1 : Constant  Value=0  OutDataTypeStr=Inherit: Inherit via back propagation
  Constant2 : Constant  OutDataTypeStr=Inherit: Inherit via back propagation
  Constant3 : Constant  Value=0  OutDataTypeStr=Inherit: Inherit via back propagation
  Constant7 : Constant  Value=StSys_stCondActv_C
  Delay : Delay  DelayLength=1  InitialCondition=0
  Delay2 : Delay  DelayLength=1  InitialCondition=0
  Logical Operator{,1..4} (5 alike) : Logic  AllPortsSameDT=off  OutDataTypeStr=boolean
  Logical Operator6 : Logic  Operator=NOT  AllPortsSameDT=off  OutDataTypeStr=boolean
  Logical Operator7 : Logic  Operator=OR  AllPortsSameDT=off  OutDataTypeStr=boolean
  Switch : Switch  Criteria=u2 ~= 0
  Switch{1..6,29,36} (8 alike) : Switch  Criteria=u2 ~= 0  InputSameDT=on
  Switch7 : Switch  Criteria=u2 ~= 0
  Switch8 : Switch  Criteria=u2 ~= 0
  StSys_stValidReq_mp : Outport
  wires:
  Switch29/1 -> Switch8/3, Delay2/1  "StSys_stValidReq_mp"
  Bit Set24/1 -> Switch29/1
  Bit Clear41/1 -> Switch29/3
  Switch36/1 -> Bit Clear41/1, Bit Set24/1
  Bit Set18/1 -> Switch36/1
  Bit Clear54/1 -> Switch36/3
  Switch1/1 -> Bit Set18/1, Bit Clear54/1
  Bit Set1/1 -> Switch1/1
  Bit Clear1/1 -> Switch1/3
  Switch2/1 -> Bit Set1/1, Bit Clear1/1
  Bit Set2/1 -> Switch2/1
  Bit Clear2/1 -> Switch2/3
  Switch3/1 -> Bit Clear2/1, Bit Set2/1
  Bit Set3/1 -> Switch3/1
  Bit Clear3/1 -> Switch3/3
  Switch4/1 -> Bit Set3/1, Bit Clear3/1
  Bit Set4/1 -> Switch4/1
  Bit Clear4/1 -> Switch4/3
  Switch5/1 -> Bit Set4/1, Bit Clear4/1
  Bit Set5/1 -> Switch5/1
  Bit Clear5/1 -> Switch5/3
  Switch6/1 -> Bit Set5/1, Bit Clear5/1
  Bit Set6/1 -> Switch6/1
  Bit Clear6/1 -> Switch6/3
  Delay2/1 -> Bit Clear6/1, Bit Set6/1
  StSys_stStrtReq_mp/1 -> Bitwise Operator4/1, Bitwise Operator3/1, Bitwise Operator2/1, Bitwise Operator1/1, Bitwise Operator/1
  Bitwise Operator/1 -> Logical Operator/2
  Bitwise Operator5/1 -> Logical Operator/1
  Bitwise Operator1/1 -> Logical Operator1/2
  Logical Operator1/1 -> Switch36/2
  Logical Operator/1 -> Switch29/2
  Constant/1 -> Switch6/2, Switch5/2, Switch4/2
  Bitwise Operator6/1 -> Logical Operator1/1
  Constant7/1 -> Bitwise Operator9/1, Bitwise Operator8/1, Bitwise Operator7/1, Bitwise Operator6/1, Bitwise Operator5/1
  Bitwise Operator7/1 -> Logical Operator2/1
  Bitwise Operator2/1 -> Logical Operator2/2
  Bitwise Operator8/1 -> Logical Operator3/1
  Bitwise Operator3/1 -> Logical Operator3/2
  Bitwise Operator9/1 -> Logical Operator4/1
  Bitwise Operator4/1 -> Logical Operator4/2
  Logical Operator2/1 -> Switch1/2
  Logical Operator3/1 -> Switch2/2
  Logical Operator4/1 -> Switch3/2
  Switch7/1 -> Switch8/2, Delay/1
  Switch/1 -> Switch7/3
  Constant1/1 -> Switch7/1
  Constant2/1 -> Switch/1
  Logical Operator7/1 -> Switch7/2
  Logical Operator6/1 -> Logical Operator7/2
  CoETS_stEngEmgcyRunReq/1 -> Logical Operator7/1
  CoETS_stEngStopReq/1 -> Switch/2, Logical Operator6/1
  Delay/1 -> Switch/3
  Constant3/1 -> Switch8/1
  Switch8/1 -> StSys_stValidReq_mp/1

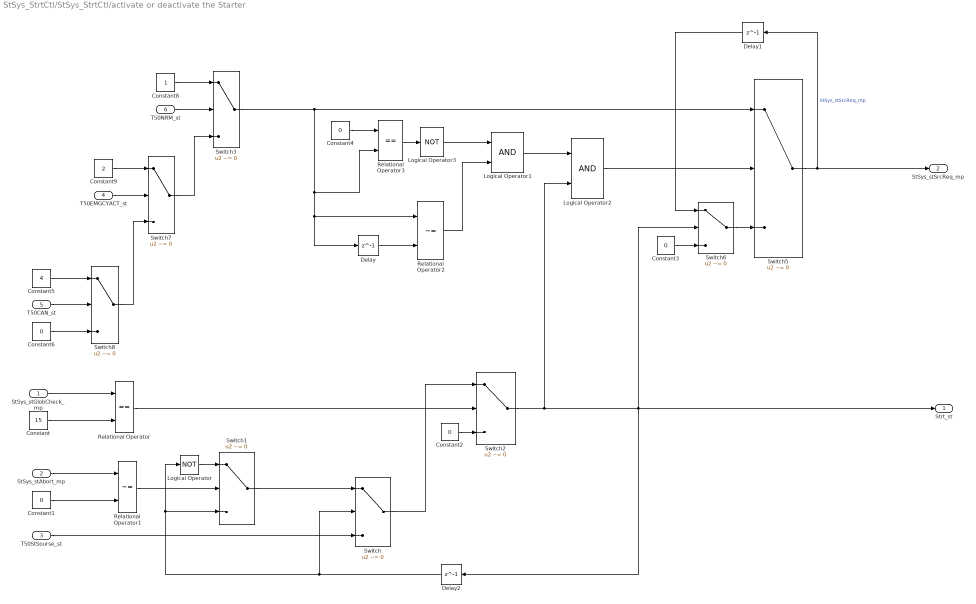
== system StSys_StrtCtl/StSys_StrtCtl/activate or deactivate the Starter ==
  StSys_stGlobCheck_mp : Inport
  StSys_stAbort_mp : Inport  Port=2
  T50StSourse_st : Inport  Port=3
  T50EMGCYACT_st : Inport  Port=4
  T50CAN_st : Inport  Port=5
  T50NRM_st : Inport  Port=6
  Constant : Constant  Value=15  OutDataTypeStr=Inherit: Inherit via back propagation
  Constant{1..4} (4 alike) : Constant  Value=0  OutDataTypeStr=Inherit: Inherit via back propagation
  Constant5 : Constant  Value=4  OutDataTypeStr=Inherit: Inherit via back propagation
  Constant6 : Constant  Value=0  OutDataTypeStr=uint8
  Constant8 : Constant  OutDataTypeStr=uint8
  Constant9 : Constant  Value=2  OutDataTypeStr=Inherit: Inherit via back propagation
  Delay : Delay  DelayLength=1  InitialCondition=0
  Delay1 : Delay  DelayLength=1  InitialCondition=0
  Delay2 : Delay  DelayLength=1  InitialCondition=0
  Logical Operator : Logic  Operator=NOT  AllPortsSameDT=off  OutDataTypeStr=boolean
  Logical Operator1 : Logic  AllPortsSameDT=off  OutDataTypeStr=boolean
  Logical Operator2 : Logic  AllPortsSameDT=off  OutDataTypeStr=boolean
  Logical Operator3 : Logic  Operator=NOT  AllPortsSameDT=off  OutDataTypeStr=boolean
  Relational Operator : RelationalOperator  Operator===  RndMeth=Simplest  InputSameDT=on
  Relational Operator1 : RelationalOperator  Operator=~=  RndMeth=Simplest  InputSameDT=on
  Relational Operator2 : RelationalOperator  Operator=~=  OutDataTypeStr=boolean  RndMeth=Simplest  InputSameDT=on
  Relational Operator3 : RelationalOperator  Operator===  OutDataTypeStr=boolean  RndMeth=Simplest  InputSameDT=on
  Switch : Switch  Criteria=u2 ~= 0
  Switch1 : Switch  Criteria=u2 ~= 0
  Switch2 : Switch  Criteria=u2 ~= 0  OutDataTypeStr=Inherit: Inherit via back propagation  InputSameDT=on
  Switch3 : Switch  Criteria=u2 ~= 0  OutDataTypeStr=Inherit: Inherit via back propagation  InputSameDT=on
  Switch5 : Switch  Criteria=u2 ~= 0
  Switch6 : Switch  Criteria=u2 ~= 0  OutDataTypeStr=Inherit: Inherit via back propagation  InputSameDT=on
  Switch7 : Switch  Criteria=u2 ~= 0  InputSameDT=on
  Switch8 : Switch  Criteria=u2 ~= 0  InputSameDT=on
  Strt_st : Outport  OutDataTypeStr=boolean
  StSys_stSrcReq_mp : Outport  Port=2
  wires:
  StSys_stGlobCheck_mp/1 -> Relational Operator/1
  Constant/1 -> Relational Operator/2
  StSys_stAbort_mp/1 -> Relational Operator1/1
  Constant1/1 -> Relational Operator1/2
  Relational Operator1/1 -> Switch1/2
  Switch2/1 -> Delay2/1, Switch6/2, Strt_st/1, Logical Operator2/2
  Relational Operator/1 -> Switch2/2
  Switch/1 -> Switch2/1
  Constant2/1 -> Switch2/3
  Switch1/1 -> Switch/1
  Logical Operator/1 -> Switch1/1
  Delay2/1 -> Switch/2, Switch1/3, Logical Operator/1
  T50StSourse_st/1 -> Switch/3
  Switch5/1 -> StSys_stSrcReq_mp/1, Delay1/1  "StSys_stSrcReq_mp"
  Delay/1 -> Relational Operator2/2
  Switch3/1 -> Delay/1, Relational Operator2/1, Relational Operator3/2, Switch5/1
  Logical Operator2/1 -> Switch5/2
  Delay1/1 -> Switch6/1
  Switch6/1 -> Switch5/3
  Constant3/1 -> Switch6/3
  Constant4/1 -> Relational Operator3/1
  Relational Operator3/1 -> Logical Operator3/1
  Relational Operator2/1 -> Logical Operator1/2
  Logical Operator1/1 -> Logical Operator2/1
  Logical Operator3/1 -> Logical Operator1/1
  T50NRM_st/1 -> Switch3/2
  Constant8/1 -> Switch3/1
  Switch7/1 -> Switch3/3
  T50EMGCYACT_st/1 -> Switch7/2
  Constant9/1 -> Switch7/1
  Switch8/1 -> Switch7/3
  T50CAN_st/1 -> Switch8/2
  Constant5/1 -> Switch8/1
  Constant6/1 -> Switch8/3

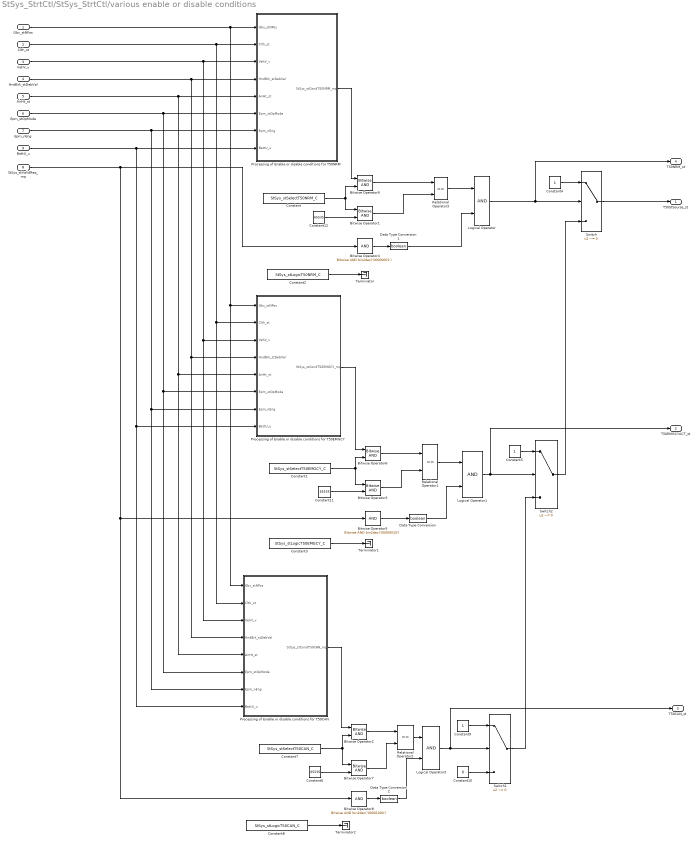
== system StSys_StrtCtl/StSys_StrtCtl/various enable or disable conditions ==
  Gbx_stNPos : Inport
  Clth_st : Inport  Port=2
  VehV_v : Inport  Port=3
  HndBrk_stDebVal : Inport  Port=4
  AirHt_st : Inport  Port=5
  Epm_stOpMode : Inport  Port=6
  Epm_nEng : Inport  Port=7
  StSys_stValidReq_mp : Inport  Port=8
  BattU_u : Inport  Port=9
  Bitwise Operator{1..3,6..7,9} (6 alike) : simulink/Logic and Bit Operations/Bitwise Operator  logicop=AND  UseBitMask=off  NumInputPorts=2  BitMask=bin2dec('11011001')  BitMaskRealWorld=Stored Integer
  Bitwise Operator4 : simulink/Logic and Bit Operations/Bitwise Operator  logicop=AND  UseBitMask=on  BitMask=bin2dec('00000001')  BitMaskRealWorld=Stored Integer
  Bitwise Operator5 : simulink/Logic and Bit Operations/Bitwise Operator  logicop=AND  UseBitMask=on  BitMask=bin2dec('00000010')  BitMaskRealWorld=Stored Integer
  Bitwise Operator8 : simulink/Logic and Bit Operations/Bitwise Operator  logicop=AND  UseBitMask=on  BitMask=bin2dec('00001000')  BitMaskRealWorld=Stored Integer
  Constant : Constant  Value=StSys_stSelectT50NRM_C
  Constant1 : Constant  Value=StSys_stSelectT50EMGCY_C
  Constant10 : Constant  Value=0  OutDataTypeStr=boolean
  Constant11 : Constant  Value=65535  OutDataTypeStr=Inherit: Inherit via back propagation
  Constant12 : Constant  Value=65535  OutDataTypeStr=Inherit: Inherit via back propagation
  Constant2 : Constant  Value=StSys_stLogicT50NRM_C
  Constant3 : Constant  Value=StSys_stLogicT50EMGCY_C
  Constant4 : Constant  OutDataTypeStr=Inherit: Inherit via back propagation
  Constant5 : Constant  OutDataTypeStr=Inherit: Inherit via back propagation
  Constant6 : Constant  Value=65535  OutDataTypeStr=Inherit: Inherit via back propagation
  Constant7 : Constant  Value=StSys_stSelectT50CAN_C
  Constant8 : Constant  Value=StSys_stLogicT50CAN_C
  Constant9 : Constant  OutDataTypeStr=Inherit: Inherit via back propagation
  Data Type Conversion : DataTypeConversion  OutDataTypeStr=boolean
  Data Type Conversion1 : DataTypeConversion  OutDataTypeStr=boolean
  Data Type Conversion2 : DataTypeConversion  OutDataTypeStr=boolean
  Logical Operator : Logic  AllPortsSameDT=off  OutDataTypeStr=boolean
  Logical Operator1 : Logic  OutDataTypeStr=boolean
  Logical Operator3 : Logic  AllPortsSameDT=off  OutDataTypeStr=boolean
  Processing of Enable or disable conditions for T50CAN : Subsystem
  Processing of Enable or disable conditions for T50EMGCY : Subsystem
  Processing of Enable or disable conditions for T50NRM : Subsystem
  Relational Operator1 : RelationalOperator  Operator===  OutDataTypeStr=boolean  RndMeth=Simplest  InputSameDT=on
  Relational Operator2 : RelationalOperator  Operator===  OutDataTypeStr=boolean  RndMeth=Simplest  InputSameDT=on
  Relational Operator3 : RelationalOperator  Operator===  OutDataTypeStr=boolean  RndMeth=Simplest
  Switch : Switch  Criteria=u2 ~= 0  InputSameDT=on
  Switch1 : Switch  Criteria=u2 ~= 0  InputSameDT=on
  Switch2 : Switch  Criteria=u2 ~= 0  InputSameDT=on
  Terminator : Terminator
  Terminator1 : Terminator
  Terminator2 : Terminator
  T50StSourse_st : Outport
  T50EMGCYACT_st : Outport  Port=2
  T50CAN_st : Outport  Port=3
  T50NRM_st : Outport  Port=4
  wires:
  Switch/1 -> T50StSourse_st/1
  Bitwise Operator4/1 -> Data Type Conversion1/1
  Bitwise Operator5/1 -> Data Type Conversion/1
  Relational Operator1/1 -> Logical Operator1/1
  Switch2/1 -> Switch/3
  Constant4/1 -> Switch/1
  Constant5/1 -> Switch2/1
  Switch1/1 -> Switch2/3
  Data Type Conversion/1 -> Logical Operator1/2
  Data Type Conversion1/1 -> Logical Operator/2
  Logical Operator1/1 -> T50EMGCYACT_st/1, Switch2/2
  Logical Operator/1 -> T50NRM_st/1, Switch/2
  Constant7/1 -> Bitwise Operator2/2, Bitwise Operator7/1
  Bitwise Operator8/1 -> Data Type Conversion2/1
  Relational Operator2/1 -> Logical Operator3/1
  Constant9/1 -> Switch1/1
  Constant10/1 -> Switch1/3
  Data Type Conversion2/1 -> Logical Operator3/2
  Logical Operator3/1 -> T50CAN_st/1, Switch1/2
  Constant1/1 -> Bitwise Operator6/2, Bitwise Operator3/1
  Relational Operator3/1 -> Logical Operator/1
  Constant/1 -> Bitwise Operator9/2, Bitwise Operator1/1
  Processing of Enable or disable conditions for T50CAN/1(StSys_stCondT50CAN_mp) -> Bitwise Operator2/1
  Constant8/1 -> Terminator2/1
  Constant6/1 -> Bitwise Operator7/2
  Bitwise Operator2/1 -> Relational Operator2/1
  Bitwise Operator7/1 -> Relational Operator2/2
  Constant3/1 -> Terminator1/1
  Constant11/1 -> Bitwise Operator3/2
  Processing of Enable or disable conditions for T50EMGCY/1(StSys_stCondT50EMGCY_mp) -> Bitwise Operator6/1
  Bitwise Operator6/1 -> Relational Operator1/1
  Bitwise Operator3/1 -> Relational Operator1/2
  Constant2/1 -> Terminator/1
  Constant12/1 -> Bitwise Operator1/2
  Processing of Enable or disable conditions for T50NRM/1(StSys_stCondT50NRM_mp) -> Bitwise Operator9/1
  Bitwise Operator9/1 -> Relational Operator3/1
  Bitwise Operator1/1 -> Relational Operator3/2
  Gbx_stNPos/1 -> Processing of Enable or disable conditions for T50EMGCY/1(Gbx_stNPos), Processing of Enable or disable conditions for T50CAN/1(Gbx_stNPos), Processing of Enable or disable conditions for T50NRM/1(Gbx_stNPos)
  Clth_st/1 -> Processing of Enable or disable conditions for T50EMGCY/2(Clth_st), Processing of Enable or disable conditions for T50CAN/2(Clth_st), Processing of Enable or disable conditions for T50NRM/2(Clth_st)
  VehV_v/1 -> Processing of Enable or disable conditions for T50CAN/3(VehV_v), Processing of Enable or disable conditions for T50EMGCY/3(VehV_v), Processing of Enable or disable conditions for T50NRM/3(VehV_v)
  HndBrk_stDebVal/1 -> Processing of Enable or disable conditions for T50CAN/4(HndBrk_stDebVal), Processing of Enable or disable conditions for T50EMGCY/4(HndBrk_stDebVal), Processing of Enable or disable conditions for T50NRM/4(HndBrk_stDebVal)
  AirHt_st/1 -> Processing of Enable or disable conditions for T50EMGCY/5(AirHt_st), Processing of Enable or disable conditions for T50CAN/5(AirHt_st), Processing of Enable or disable conditions for T50NRM/5(AirHt_st)
  Epm_stOpMode/1 -> Processing of Enable or disable conditions for T50CAN/6(Epm_stOpMode), Processing of Enable or disable conditions for T50EMGCY/6(Epm_stOpMode), Processing of Enable or disable conditions for T50NRM/6(Epm_stOpMode)
  Epm_nEng/1 -> Processing of Enable or disable conditions for T50CAN/7(Epm_nEng), Processing of Enable or disable conditions for T50EMGCY/7(Epm_nEng), Processing of Enable or disable conditions for T50NRM/7(Epm_nEng)
  BattU_u/1 -> Processing of Enable or disable conditions for T50CAN/8(BattU_u), Processing of Enable or disable conditions for T50EMGCY/8(BattU_u), Processing of Enable or disable conditions for T50NRM/8(BattU_u)
  StSys_stValidReq_mp/1 -> Bitwise Operator8/1, Bitwise Operator5/1, Bitwise Operator4/1
